simulink model "BackStepping_ex1_2"  (R2021a)
settings: Solver=VariableStepAuto  StartTime=0.0  StopTime=30  RelTol=1e-3
settings Model: Creator=JianFongLee  LastModifiedBy=JianFongLee

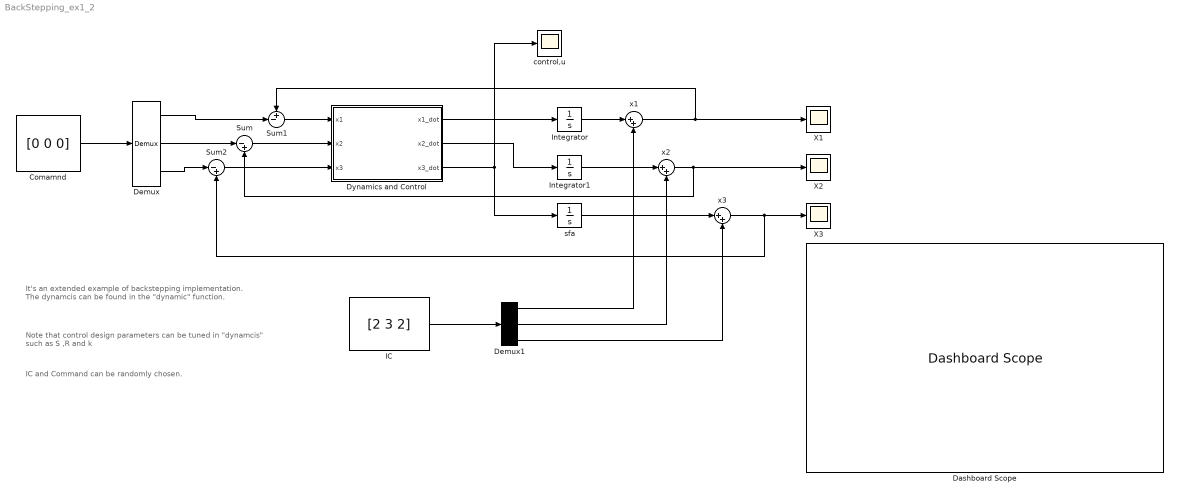
== system BackStepping_ex1_2 ==
  note: IC and Command can be randomly chosen.
  note: Note that control design parameters can be tuned in "dynamcis"
      | such as S ,R and k
  note: It's an extended example of backstepping implementation.
      | The dynamcis can be found in the "dynamic" function.
  Comamnd : Constant  Value=[0 0 0]
  Dashboard Scope : DashboardScope
  Demux : Demux  Outputs=3
      settings: DisplayOption=none
  Demux1 : Demux  Outputs=3
      settings: DisplayOption=none
  Dynamics and Control : MATLAB Function  TreatAsAtomicUnit=on
  IC : Constant  Value=[2 3 2]
  Integrator : Integrator
  Integrator1 : Integrator
  Sum : Sum  Inputs=|-+
  Sum1 : Sum  Inputs=+-|
  Sum2 : Sum  Inputs=|-+
  X1 : Scope
  X2 : Scope
  X3 : Scope
  control,u : Scope
  sfa : Integrator
  x1 : Sum  Inputs=|++
  x2 : Sum  Inputs=|++
  x3 : Sum  Inputs=|++
  wires:
  Dynamics and Control/1(x1_dot) -> Integrator/1
  Dynamics and Control/2(x2_dot) -> Integrator1/1
  Sum/1 -> Dynamics and Control/2(x2)
  Sum1/1 -> Dynamics and Control/1(x1)
  IC/1 -> Demux1/1
  Demux1/1 -> x1/2
  Integrator/1 -> x1/1
  x1/1 -> Sum1/1, X1/1
  Integrator1/1 -> x2/1
  x2/1 -> X2/1, Sum/2
  Demux1/2 -> x2/2
  Sum2/1 -> Dynamics and Control/3(x3)
  x3/1 -> X3/1, Sum2/2
  Dynamics and Control/3(x3_dot) -> sfa/1, control,u/1
  sfa/1 -> x3/1
  Demux1/3 -> x3/2
  Comamnd/1 -> Demux/1
  Demux/3 -> Sum2/1
  Demux/2 -> Sum/1
  Demux/1 -> Sum1/2

== matlab function BackStepping_ex1_2/Dynamics and Control ==
  data: x1 input; x1_dot output; x2 input; x2_dot output; x3 input; x3_dot output
function [x1_dot,x2_dot, x3_dot]= dynamics(x1, x2, x3)
x1_Dum= x1^2 - x1^3 + x2;  %%% Dunmmy for the Dynamics of x1_dot

%%% Parameters determination
k = 2.7; %%% Choose k > 0 
S = 1;   %%% S == 1 is the sweetspot
R = 10;  %% Maximum output of u

%%% Control u here
P = x1 + 2*x1^3 - 2*x1^4 + 2*x1*x2;
P_dot = x1_Dum * (1 + 6*x1^2 - 8*x1^3 + 2*x2) + 2*x1*x3;
u = -1*P_dot - x2 - x1^2 - k*(x3+P)^S;

%%% Add a control restriction
if abs(u) > abs(R)
   if u>0
       u = abs(R);
   else
       u = -1*abs(R);
   end
end

%%% Compute dynamics
x1_dot = x1_Dum;              %%% Dynamics of x1_dot
x2_dot = x3;                %%% Dynamics of x2_dot
x3_dot = u;                 %%% Dynamics of x3_dot


%%% Lynapunov functions
%%% V = 0.5*x1^2 + 0.5*(x1+x2^2)^2 + 0.5*(x3+P)^2;

%%% Notation on S, the power determines how radical V_dot is
%%% S therotically could be any odd greater than 0,
%%% but experiments show that S = 3 or 5 would lead to significant oscillation
